simulink model "eksperyment"  (R2017a)
settings: Solver=ode45  StartTime=0.0  StopTime=100  MaxStep=0.1  MinStep=0.01  RelTol=1e-2  EnableMultiTasking=on
undefined symbols (not defined in the file or in its folder): A0, A120, A150, A180, A30, A60, A90, B0, B120, B150, B180, B30, B60, B90
libraries: fuzblock x1
settings Model: Creator=student  LastModifiedBy=Szwank
settings OptimizationCC: LifeSpan=inf
settings DebuggingCC: SFUnexpectedBacktrackingDiag=warning  SFNoUnconditionalDefaultTransitionDiag=warning  SFExecutionAtInitializationDiag=none
settings GRTTargetCC: TargetLangStandard=C89/C90 (ANSI)  GeneratePreprocessorConditionals=Disable all
settings ConfigComp: CovMetricSettings=dw  CovHtmlReporting=on  CovSaveCumulativeToWorkspaceVar=on  CovSaveSingleToWorkspaceVar=on  CovExternalEMLEnable=off

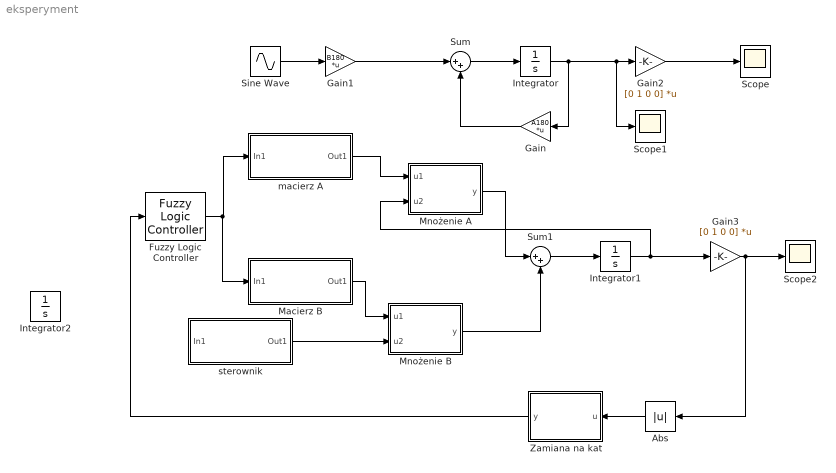
== system eksperyment ==
  Abs : Abs
  Fuzzy Logic Controller : fuzblock/Fuzzy Logic  Controller  fis=['modelRozmyty.fis']
  Gain : Gain  Gain=A180  Multiplication=Matrix(K*u)
  Gain1 : Gain  Gain=B180  Multiplication=Matrix(K*u)
  Gain2 : Gain  Gain=[0 1 0 0]  Multiplication=Matrix(K*u)
  Gain3 : Gain  Gain=[0 1 0 0]  Multiplication=Matrix(K*u)
  Integrator : Integrator  InitialCondition=[0 pi+0.1 0 0]
  Integrator1 : Integrator  InitialCondition=[0 pi+0.1 0 0]
  Integrator2 : Integrator  InitialCondition=[0 pi+0.1 0 0]
  Macierz B : Subsystem
  "Mnożenie A " : MATLAB Function  TreatAsAtomicUnit=on
  "Mnożenie B " : MATLAB Function  TreatAsAtomicUnit=on
  Scope : Scope
  Scope1 : Scope
  Scope2 : Scope
  Sine Wave : Sin  Amplitude=0.1  SampleTime=0
  Sum : Sum  Inputs=|++
  Sum1 : Sum  Inputs=|++
  Zamiana na kat : MATLAB Function  TreatAsAtomicUnit=on
  "macierz A " : Subsystem
  "sterownik " : Subsystem
  wires:
  Gain/1 -> Sum/2
  Sum/1 -> Integrator/1
  Gain1/1 -> Sum/1
  Integrator/1 -> Scope1/1, Gain2/1, Gain/1
  Gain2/1 -> Scope/1
  Sine Wave/1 -> Gain1/1
  Fuzzy Logic Controller/1 -> Macierz B/1(In1), "macierz A "/1(In1)
  "macierz A "/1(Out1) -> "Mnożenie A "/1(u1)
  Sum1/1 -> Integrator1/1
  Integrator1/1 -> Gain3/1, "Mnożenie A "/2(u2)
  "Mnożenie A "/1(y) -> Sum1/1
  Macierz B/1(Out1) -> "Mnożenie B "/1(u1)
  "Mnożenie B "/1(y) -> Sum1/2
  Gain3/1 -> Abs/1, Scope2/1
  Abs/1 -> Zamiana na kat/1(u)
  Zamiana na kat/1(y) -> Fuzzy Logic Controller/1
  "sterownik "/1(Out1) -> "Mnożenie B "/2(u2)

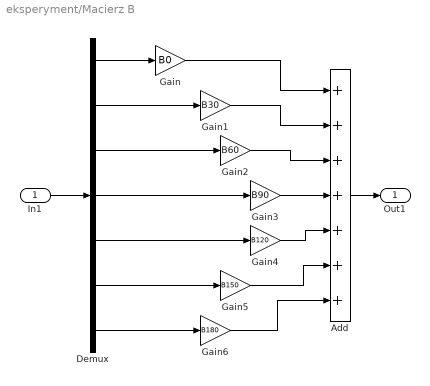
== system eksperyment/Macierz B ==
  In1 : Inport
  Add : Sum  Inputs=+++++++
  Demux : Demux  Outputs=7
  Gain : Gain  Gain=B0
  Gain1 : Gain  Gain=B30
  Gain2 : Gain  Gain=B60
  Gain3 : Gain  Gain=B90
  Gain4 : Gain  Gain=B120
  Gain5 : Gain  Gain=B150
  Gain6 : Gain  Gain=B180
  Out1 : Outport
  wires:
  In1/1 -> Demux/1
  Demux/2 -> Gain1/1
  Demux/3 -> Gain2/1
  Demux/1 -> Gain/1
  Demux/4 -> Gain3/1
  Demux/5 -> Gain4/1
  Demux/6 -> Gain5/1
  Demux/7 -> Gain6/1
  Gain/1 -> Add/1
  Gain1/1 -> Add/2
  Gain2/1 -> Add/3
  Gain3/1 -> Add/4
  Gain4/1 -> Add/5
  Gain5/1 -> Add/6
  Gain6/1 -> Add/7
  Add/1 -> Out1/1

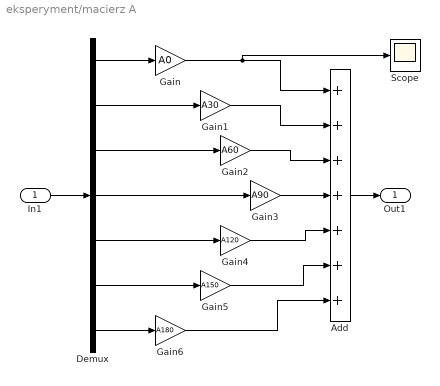
== system eksperyment/macierz A  ==
  In1 : Inport
  Add : Sum  Inputs=+++++++
  Demux : Demux  Outputs=7
  Gain : Gain  Gain=A0
  Gain1 : Gain  Gain=A30
  Gain2 : Gain  Gain=A60
  Gain3 : Gain  Gain=A90
  Gain4 : Gain  Gain=A120
  Gain5 : Gain  Gain=A150
  Gain6 : Gain  Gain=A180
  Scope : Scope
  Out1 : Outport
  wires:
  In1/1 -> Demux/1
  Demux/2 -> Gain1/1
  Demux/3 -> Gain2/1
  Demux/1 -> Gain/1
  Demux/4 -> Gain3/1
  Demux/5 -> Gain4/1
  Demux/6 -> Gain5/1
  Demux/7 -> Gain6/1
  Gain/1 -> Scope/1, Add/1
  Gain1/1 -> Add/2
  Gain2/1 -> Add/3
  Gain3/1 -> Add/4
  Gain4/1 -> Add/5
  Gain5/1 -> Add/6
  Gain6/1 -> Add/7
  Add/1 -> Out1/1

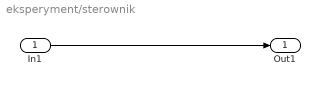
== system eksperyment/sterownik  ==
  In1 : Inport
  Out1 : Outport
  wires:
  In1/1 -> Out1/1

== matlab function eksperyment/Mnożenie B  ==
  data: u1 input; y output; u2 input
function y = fcn(u1,u2)

y = u1*u2;

== matlab function eksperyment/Mnożenie A  ==
  data: u1 input; y output; u2 input
function y = fcn(u1,u2)

y = u1*u2;

== matlab function eksperyment/Zamiana na kat ==
  data: u input; y output
function y = fcn(u)

g=u*180/pi;
if(g>180)
    reszta=rem(g,180);
    if(rem(fix(g/180),2)==1)
        g=180-reszta;
    else
        g=reszta;
    end

end
y = g;
